simulink model "exp1"  (R2020b)
settings: Solver=VariableStepAuto  StartTime=0.0  StopTime=40  RelTol=1e-3
libraries: simulink x2
settings Model: Creator=suryanshshukla  LastModifiedBy=suryanshshukla

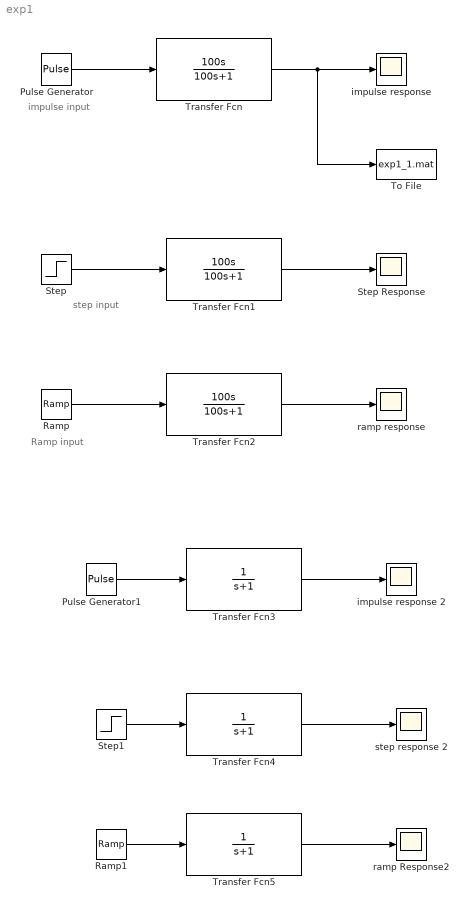
== system exp1 ==
  note: impulse input
  note: Ramp input
  note: step input
  Pulse Generator : DiscretePulseGenerator  PulseType=Time based  Period=10  PulseWidth=5
  Pulse Generator1 : DiscretePulseGenerator  PulseType=Time based  Period=10  PulseWidth=5
  Ramp : simulink/Sources/Ramp  slope=1  start=0  InitialOutput=0
  Ramp1 : simulink/Sources/Ramp  slope=1  start=0  InitialOutput=0
  Step : Step  SampleTime=0
  Step Response : Scope
  Step1 : Step  SampleTime=0
  To File : ToFile  Filename=exp1_1.mat  SaveFormat=Timeseries
  Transfer Fcn : TransferFcn  Numerator=[100,0]  Denominator=[100,1]
  Transfer Fcn1 : TransferFcn  Numerator=[100,0]  Denominator=[100,1]
  Transfer Fcn2 : TransferFcn  Numerator=[100,0]  Denominator=[100,1]
  Transfer Fcn3 : TransferFcn  Denominator=[1,1]
  Transfer Fcn4 : TransferFcn  Denominator=[1,1]
  Transfer Fcn5 : TransferFcn  Denominator=[1,1]
  impulse response : Scope
  impulse response 2 : Scope
  ramp Response2 : Scope
  ramp response : Scope
  step response 2 : Scope
  wires:
  Pulse Generator/1 -> Transfer Fcn/1
  Transfer Fcn/1 -> To File/1, impulse response/1
  Step/1 -> Transfer Fcn1/1
  Ramp/1 -> Transfer Fcn2/1
  Transfer Fcn1/1 -> Step Response/1
  Transfer Fcn2/1 -> ramp response/1
  Pulse Generator1/1 -> Transfer Fcn3/1
  Transfer Fcn3/1 -> impulse response 2/1
  Step1/1 -> Transfer Fcn4/1
  Ramp1/1 -> Transfer Fcn5/1
  Transfer Fcn5/1 -> ramp Response2/1
  Transfer Fcn4/1 -> step response 2/1
